simulink library "SeatMdSwtchArbt_Lib"  (R2018b)
settings: Solver=VariableStepAuto  StartTime=0.0  StopTime=10.0  RelTol=1e-3
settings Model: Creator=s69u2m  LastModifiedBy=su3dcu

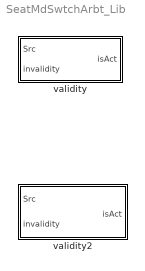
== system SeatMdSwtchArbt_Lib ==
  validity : Subsystem
  validity2 : Subsystem

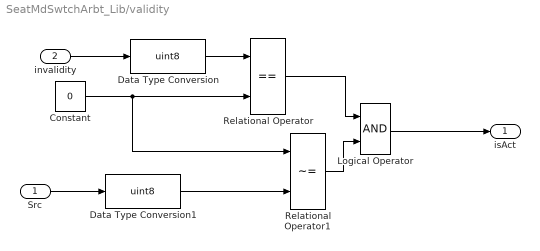
== system SeatMdSwtchArbt_Lib/validity ==
  Src : Inport
  invalidity : Inport  Port=2
  Constant : Constant  Value=0  OutDataTypeStr=uint8
  Data Type Conversion : DataTypeConversion  OutDataTypeStr=uint8
  Data Type Conversion1 : DataTypeConversion  OutDataTypeStr=uint8
  Logical Operator : Logic  AllPortsSameDT=off  OutDataTypeStr=boolean
  Relational Operator : RelationalOperator  Operator===  OutDataTypeStr=boolean  RndMeth=Simplest
  Relational Operator1 : RelationalOperator  Operator=~=  OutDataTypeStr=boolean  RndMeth=Simplest
  isAct : Outport
  wires:
  invalidity/1 -> Data Type Conversion/1
  Constant/1 -> Relational Operator1/1, Relational Operator/2
  Data Type Conversion/1 -> Relational Operator/1
  Relational Operator/1 -> Logical Operator/1
  Logical Operator/1 -> isAct/1
  Data Type Conversion1/1 -> Relational Operator1/2
  Src/1 -> Data Type Conversion1/1
  Relational Operator1/1 -> Logical Operator/2

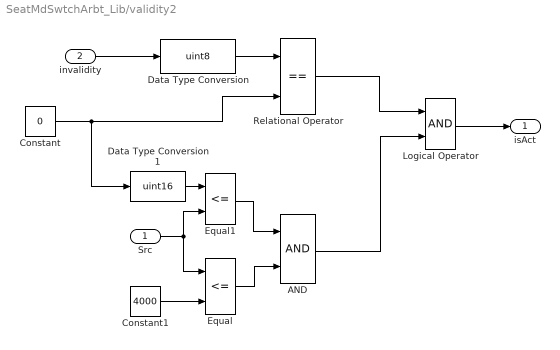
== system SeatMdSwtchArbt_Lib/validity2 ==
  Src : Inport
  invalidity : Inport  Port=2
  AND : Logic  AllPortsSameDT=off  OutDataTypeStr=boolean
  Constant : Constant  Value=0  OutDataTypeStr=uint8
  Constant1 : Constant  Value=4000  OutDataTypeStr=uint16
  Data Type Conversion : DataTypeConversion  OutDataTypeStr=uint8
  Data Type Conversion1 : DataTypeConversion  OutDataTypeStr=uint16
  Equal : RelationalOperator  Operator=<=  OutDataTypeStr=boolean  RndMeth=Simplest
  Equal1 : RelationalOperator  Operator=<=  OutDataTypeStr=boolean  RndMeth=Simplest
  Logical Operator : Logic  AllPortsSameDT=off  OutDataTypeStr=boolean
  Relational Operator : RelationalOperator  Operator===  OutDataTypeStr=boolean  RndMeth=Simplest
  isAct : Outport
  wires:
  Logical Operator/1 -> isAct/1
  Data Type Conversion/1 -> Relational Operator/1
  Constant/1 -> Relational Operator/2, Data Type Conversion1/1
  Relational Operator/1 -> Logical Operator/1
  invalidity/1 -> Data Type Conversion/1
  Constant1/1 -> Equal/2
  Src/1 -> Equal/1, Equal1/2
  Data Type Conversion1/1 -> Equal1/1
  Equal/1 -> AND/2
  Equal1/1 -> AND/1
  AND/1 -> Logical Operator/2
